simulink model "Final R2022"  (R2022b)
settings: Solver=VariableStepAuto  StartTime=0.0  StopTime=10  RelTol=1e-3
libraries: dsparch4 x1, commdigbbndpm3 x1, commfilt2 x1, commrandsrc3 x1, dspsrcs4 x1
settings Model: Creator=kourosh  LastModifiedBy=kourosh
settings OptimizationCC: ReuseModelBlockBuffer=on

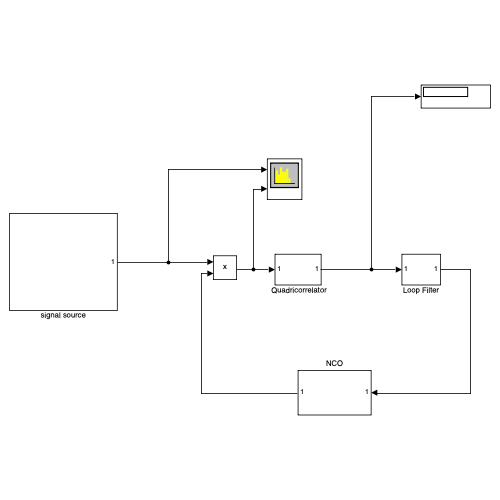
[thumbnail: Simulink's stored preview of the top-level diagram]
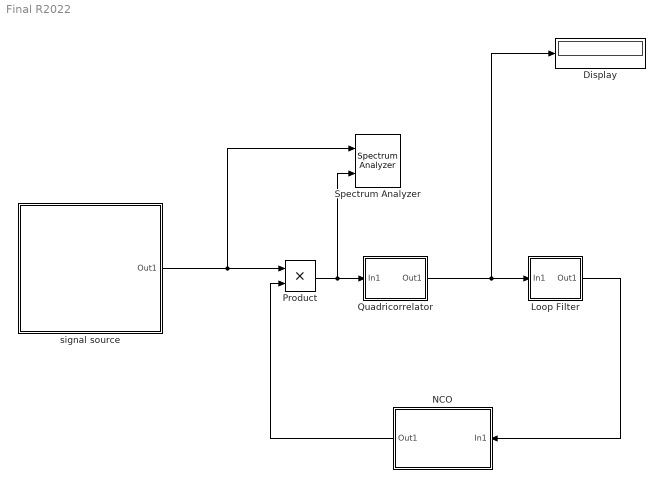
== system Final R2022 ==
  " Quadricorrelator" : Subsystem
  Display : Display
  Loop Filter : Subsystem
  NCO : Subsystem
  Product : Product
  Spectrum Analyzer : SpectrumAnalyzer  NumInputPorts=2  DefaultConfigurationName=spbscopes.SpectrumAnalyzerBlockCfg
  signal source : Subsystem
  wires:
  Product/1 -> Spectrum Analyzer/2, " Quadricorrelator"/1(In1)
  NCO/1(Out1) -> Product/2
  " Quadricorrelator"/1(Out1) -> Display/1, Loop Filter/1(In1)
  signal source/1(Out1) -> Spectrum Analyzer/1, Product/1
  Loop Filter/1(Out1) -> NCO/1(In1)

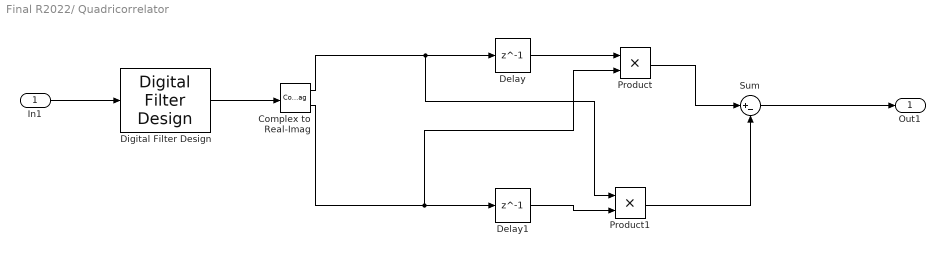
== system Final R2022/ Quadricorrelator ==
  In1 : Inport
  Complex to Real-Imag : ComplexToRealImag
  Delay : Delay  DelayLength=1
  Delay1 : Delay  DelayLength=1
  Digital Filter Design : dsparch4/Digital Filter Design  mwdsp_browser_bugfix_var=off
  Product : Product
  Product1 : Product
  Sum : Sum  Inputs=|+-
  Out1 : Outport
  wires:
  In1/1 -> Digital Filter Design/1
  Digital Filter Design/1 -> Complex to Real-Imag/1
  Complex to Real-Imag/1 -> Product1/1, Delay/1
  Complex to Real-Imag/2 -> Product/2, Delay1/1
  Sum/1 -> Out1/1
  Product1/1 -> Sum/2
  Delay1/1 -> Product1/2
  Delay/1 -> Product/1
  Product/1 -> Sum/1

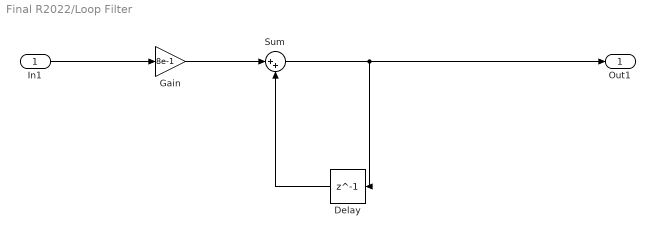
== system Final R2022/Loop Filter ==
  In1 : Inport
  Delay : Delay  DelayLength=1
  Gain : Gain  Gain=8e-1
  Sum : Sum  Inputs=|++
  Out1 : Outport
  wires:
  In1/1 -> Gain/1
  Gain/1 -> Sum/1
  Delay/1 -> Sum/2
  Sum/1 -> Delay/1, Out1/1

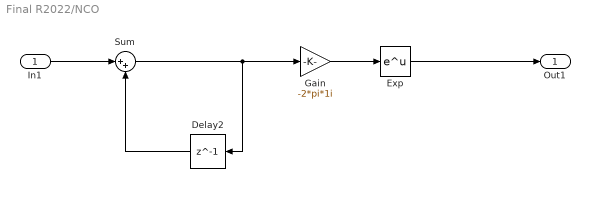
== system Final R2022/NCO ==
  In1 : Inport
  Delay2 : Delay  DelayLength=1
  Exp : Math
  Gain : Gain  Gain=-2*pi*1i
  Sum : Sum  Inputs=|++
  Out1 : Outport
  wires:
  In1/1 -> Sum/1
  Delay2/1 -> Sum/2
  Exp/1 -> Out1/1
  Gain/1 -> Exp/1
  Sum/1 -> Delay2/1, Gain/1

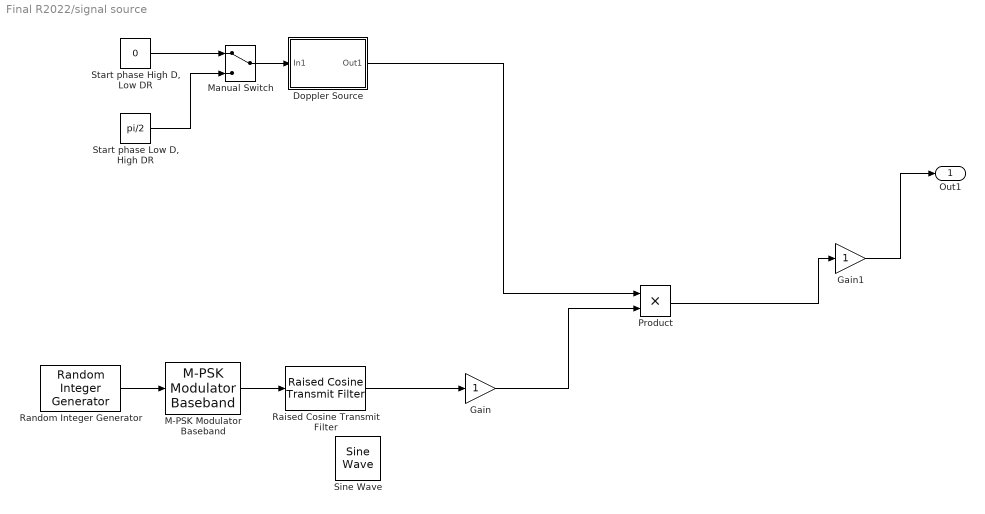
== system Final R2022/signal source ==
  Doppler Source : Subsystem
  Gain : Gain
  Gain1 : Gain
  M-PSK Modulator Baseband : commdigbbndpm3/M-PSK Modulator Baseband  M=4  InType=Integer  Enc=Gray  Mapping=[0:7]  Ph=0  outDtype=double  outWordLen=16  outUDDataType=sfix(16)  outFracLenMode=Best precision  outFracLen=15  outDataTypeStr=double  outLastDataTypeStr=double
  Manual Switch : ManualSwitch
  Product : Product
  Raised Cosine Transmit Filter : commfilt2/Raised Cosine Transmit Filter  filtType=Square root  R=0.4  filtSpan=20  N=8  filterGain=1  RateOptions=Allow multirate processing  framing=Mute  checkCoeff=off  variableName=rcTxFilt  checkGain=Normalized  sampMode=Mute  saveAsFlag=0  currentFiltSpan=20  D=(20)/2  launchFVT=on  roundingMode=Floor  overflowMode=off  coeffDataTypeStr=Inherit: Same word length as input  coeffMin=[]  coeffMax=[]  coeffLastDataTypeStr=Inherit: Same word length as input  outputDataTypeStr=Inherit: Same as accumulator  outputMin=[]  outputMax=[]  outputLastDataTypeStr=Inherit: Same as accumulator
  Random Integer Generator : commrandsrc3/Random Integer Generator  SetSize=4  SeedSource=Auto  Seed=0  SampleTime=1/50000  SamplesPerFrame=1  OutputDataType=double  SimulateUsing=Interpreted execution
  Sine Wave : dspsrcs4/Sine Wave  Amplitude=1  Frequency=50e3  Phase=0  SampleMode=Discrete  OutComplex=Complex  CompMethod=Trigonometric fcn  TableSize=Speed  SampleTime=1/(50e3*8)  SamplesPerFrame=1  ResetState=Restart at time zero  OutputFrames=off  dataType=double  wordLen=16  udDataType=sfix(16)  fracBitsMode=Best precision  numFracBits=15  OutDataTypeStr=double  LastOutDataTypeStr=double
  "Start phase High D, Low DR" : Constant  Value=0  SampleTime=1/(50e3*8)
  "Start phase Low D, High DR" : Constant  Value=pi/2  SampleTime=1/(50e3*8)
  Out1 : Outport
  wires:
  "Start phase Low D, High DR"/1 -> Manual Switch/2
  "Start phase High D, Low DR"/1 -> Manual Switch/1
  Manual Switch/1 -> Doppler Source/1(In1)
  Doppler Source/1(Out1) -> Product/1
  Random Integer Generator/1 -> M-PSK Modulator Baseband/1
  M-PSK Modulator Baseband/1 -> Raised Cosine Transmit Filter/1
  Raised Cosine Transmit Filter/1 -> Gain/1
  Gain/1 -> Product/2
  Product/1 -> Gain1/1
  Gain1/1 -> Out1/1

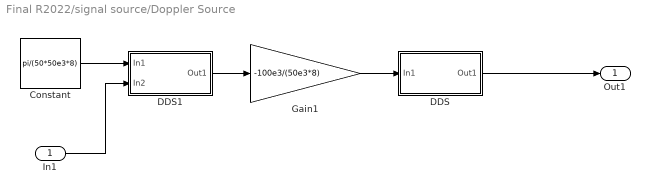
== system Final R2022/signal source/Doppler Source ==
  In1 : Inport
  Constant : Constant  Value=pi/(50*50e3*8)  SampleTime=1/(50e3*8)
  DDS : Subsystem
  DDS1 : Subsystem
  Gain1 : Gain  Gain=-100e3/(50e3*8)
  Out1 : Outport
  wires:
  In1/1 -> DDS1/2(In2)
  DDS1/1(Out1) -> Gain1/1
  Gain1/1 -> DDS/1(In1)
  Constant/1 -> DDS1/1(In1)
  DDS/1(Out1) -> Out1/1

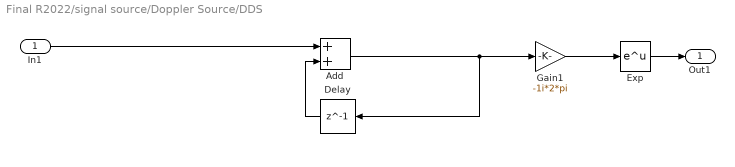
== system Final R2022/signal source/Doppler Source/DDS ==
  In1 : Inport
  Add : Sum
  Delay : Delay  DelayLength=1  SampleTime=1/(50e3*8)
  Exp : Math
  Gain1 : Gain  Gain=-1i*2*pi
  Out1 : Outport
  wires:
  Delay/1 -> Add/2
  Add/1 -> Gain1/1, Delay/1
  Exp/1 -> Out1/1
  Gain1/1 -> Exp/1
  In1/1 -> Add/1

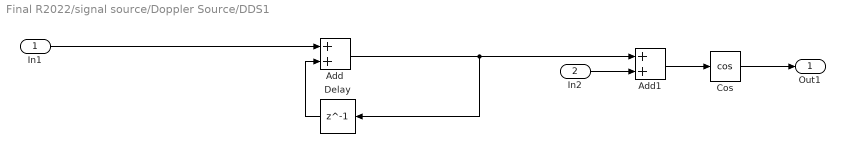
== system Final R2022/signal source/Doppler Source/DDS1 ==
  In1 : Inport
  In2 : Inport  Port=2
  Add : Sum
  Add1 : Sum
  Cos : Trigonometry  Operator=cos
  Delay : Delay  DelayLength=1  SampleTime=1/(50e3*8)
  Out1 : Outport
  wires:
  In2/1 -> Add1/2
  Add1/1 -> Cos/1
  Add/1 -> Delay/1, Add1/1
  In1/1 -> Add/1
  Cos/1 -> Out1/1
  Delay/1 -> Add/2
